simulink model "Buck_Boost_Converter_Mathematical_Model"  (R2015a)
settings: Solver=ode45  StartTime=0.0  StopTime=2  RelTol=1e-3
values from neighbouring files (symbols this model uses):
  C = 8200e-06    (= 0.0082)    [Buck_Boost_Converter_Script.m]
  fs = 200e03    (= 200000)    [Buck_Boost_Converter_Script.m]
  L = 2.2e-04    (= 0.00022)    [Buck_Boost_Converter_Script.m]
  Rm = 5.1    [Buck_Boost_Converter_Script.m]
settings Model: Creator=Koustubh  LastModifiedBy=Koustubh

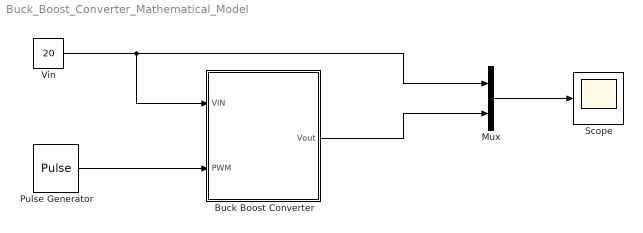
== system Buck_Boost_Converter_Mathematical_Model ==
  Buck Boost Converter : Subsystem
  Mux : Mux  Inputs=2
  Pulse Generator : DiscretePulseGenerator  PulseType=Time based  Period=1/fs  PulseWidth=0.3*100
  Scope : Scope
  Vin : Constant  Value=20
  wires:
  Vin/1 -> Buck Boost Converter/1(VIN), Mux/1
  Pulse Generator/1 -> Buck Boost Converter/2(PWM)
  Buck Boost Converter/1(Vout) -> Mux/2
  Mux/1 -> Scope/1

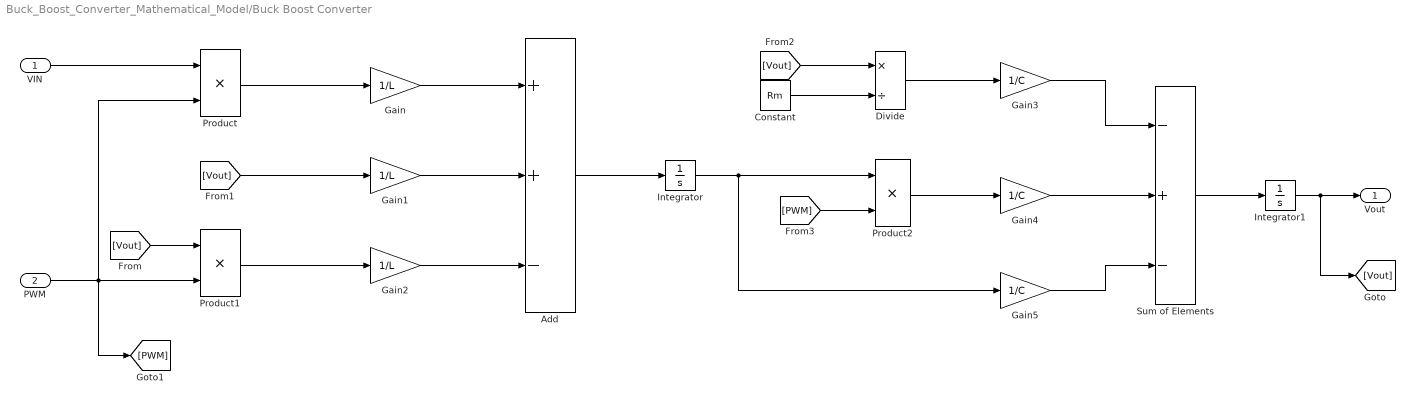
== system Buck_Boost_Converter_Mathematical_Model/Buck Boost Converter ==
  VIN : Inport
  PWM : Inport  Port=2
  Add : Sum  Inputs=++-
  Constant : Constant  Value=Rm
  Divide : Product  Inputs=*/
  Gain : Gain  Gain=1/L
  Gain1 : Gain  Gain=1/L
  Gain2 : Gain  Gain=1/L
  Gain3 : Gain  Gain=1/C
  Gain4 : Gain  Gain=1/C
  Gain5 : Gain  Gain=1/C
  Integrator : Integrator
  Integrator1 : Integrator
  Product : Product
  Product1 : Product
  Product2 : Product
  Sum of Elements : Sum  Inputs=-+-
  Vout : Outport
  wires:
  PWM/1 -> Product/2, [PWM], Product1/2
  VIN/1 -> Product/1
  Product/1 -> Gain/1
  Product1/1 -> Gain2/1
  [Vout] -> Gain1/1
  Gain2/1 -> Add/3
  Gain/1 -> Add/1
  Gain1/1 -> Add/2
  Add/1 -> Integrator/1
  Constant/1 -> Divide/2
  [Vout] -> Divide/1
  Integrator/1 -> Gain5/1, Product2/1
  [PWM] -> Product2/2
  Divide/1 -> Gain3/1
  Product2/1 -> Gain4/1
  Gain5/1 -> Sum of Elements/3
  Gain4/1 -> Sum of Elements/2
  Gain3/1 -> Sum of Elements/1
  Sum of Elements/1 -> Integrator1/1
  Integrator1/1 -> [Vout], Vout/1
  [Vout] -> Product1/1
